simulink model "RoboNouMiChi"  (R2017b)
settings: Solver=VariableStepAuto  StartTime=0.0  StopTime=10.0  RelTol=1e-3
libraries: rptgenlib x2
settings Model: Creator=prave  LastModifiedBy=prave

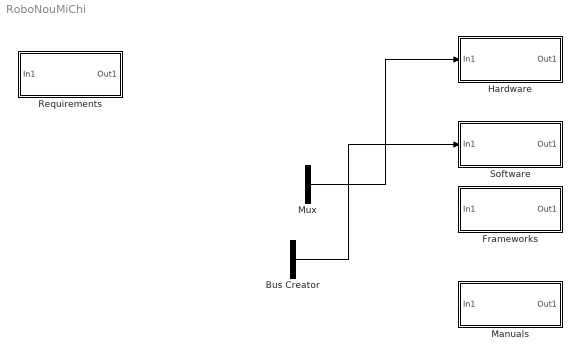
== system RoboNouMiChi ==
  Bus Creator : BusCreator  Inputs=2
  Frameworks : Subsystem  mask{Parameter1=0, Parameter2=on, Parameter3=on, Parameter4=on, Parameter5=on, Parameter6=on, Parameter7=on, Parameter8=on}
      mask prompts: Parameter1 "Heart"; Parameter2 "Heart beat estimator"; Parameter3 "Sensorless"; Parameter4 "Automotive"; Parameter5 "White balance estimator"; Parameter6 "Defect detector"; Parameter7 "Renesas"; Parameter8 "Fujitsu"
      mask DialogControl Container5 Prompt: Human
      mask DialogControl Container6 Prompt: Selection table
  Hardware : Subsystem  mask{Parameter1=0, Parameter2=on, Parameter3=on, Parameter4=on, Parameter5=on, Parameter6=on, Parameter7=on, Parameter8=on}
      mask prompts: Parameter1 "Frequency"; Parameter2 "Embedded DSP"; Parameter3 "Arm"; Parameter4 "FPGA"; Parameter5 "Cloud/Local PC"; Parameter6 "Cloud DSP"; Parameter7 "Renesas"; Parameter8 "Fujitsu"
      mask DialogControl Container5 Prompt: Hardware
      mask DialogControl Container6 Prompt: Selection table
  Manuals : Subsystem  mask{Parameter1=0, Parameter2=on, Parameter3=on, Parameter4=on, Parameter5=on, Parameter6=on, Parameter7=on, Parameter8=on}
      mask prompts: Parameter1 "Heart"; Parameter2 "Heart beat estimator"; Parameter3 "Sensorless"; Parameter4 "Automotive"; Parameter5 "White balance estimator"; Parameter6 "Defect detector"; Parameter7 "Renesas"; Parameter8 "Fujitsu"
      mask DialogControl Container5 Prompt: Human
      mask DialogControl Container6 Prompt: Selection table
  Mux : Mux  Inputs=2
  Requirements : Subsystem
  Software : Subsystem  mask{Parameter1=on, Parameter2=small, Parameter3=0}
      mask prompts: Parameter1 "Embed"; Parameter2 "C++"; Parameter3 "Frequency"
      mask TypeOptions Parameter2: small | big | medium
  wires:
  Mux/1 -> Hardware/1(In1)
  Bus Creator/1 -> Software/1(In1)

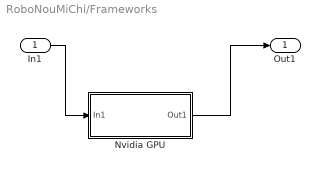
== system RoboNouMiChi/Frameworks ==
  In1 : Inport
  "Nvidia GPU " : Subsystem  TreatAsAtomicUnit=on
  Out1 : Outport
  wires:
  "Nvidia GPU "/1(Out1) -> Out1/1
  In1/1 -> "Nvidia GPU "/1(In1)

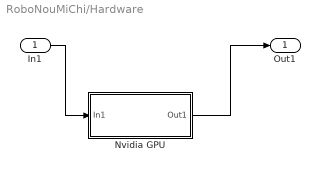
== system RoboNouMiChi/Hardware ==
  In1 : Inport
  "Nvidia GPU " : Subsystem  TreatAsAtomicUnit=on
  Out1 : Outport
  wires:
  In1/1 -> "Nvidia GPU "/1(In1)
  "Nvidia GPU "/1(Out1) -> Out1/1

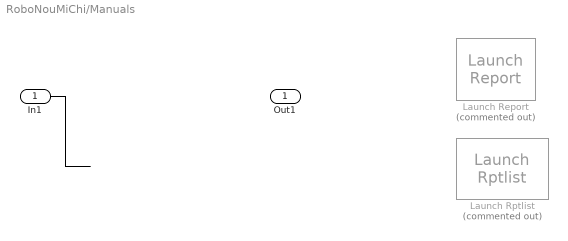
== system RoboNouMiChi/Manuals ==
  In1 : Inport
  Launch Report : rptgenlib/Launch Report  Tag=rptgen_sl  Description=Reports on the current system or model  Commented=on
      settings: SourceProductName=Simulink Report Generator  SourceProductBaseCode=SR
  Launch Rptlist : rptgenlib/Launch Rptlist  Tag=rptgen_sl  Description="This block launches the Report Generator Explorer. It lists all the setup files which the Report Generator can use to generate reports.  This GUI can also be used to set the current system's \"ReportName\" property."  Commented=on
      settings: SourceProductName=Simulink Report Generator  SourceProductBaseCode=SR
  Out1 : Outport
  wires:
  In1/1 -> ?
  ? -> Out1/1

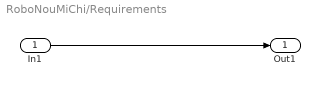
== system RoboNouMiChi/Requirements ==
  In1 : Inport
  Out1 : Outport
  wires:
  In1/1 -> Out1/1

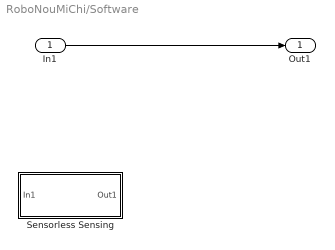
== system RoboNouMiChi/Software ==
  In1 : Inport
  "Sensorless Sensing " : Subsystem  TreatAsAtomicUnit=on
  Out1 : Outport
  wires:
  In1/1 -> Out1/1

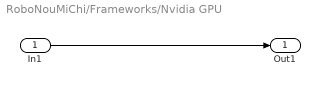
== system RoboNouMiChi/Frameworks/Nvidia GPU  ==
  In1 : Inport
  Out1 : Outport
  wires:
  In1/1 -> Out1/1

== system RoboNouMiChi/Hardware/Nvidia GPU  ==
  In1 : Inport
  Out1 : Outport
  wires:
  In1/1 -> Out1/1

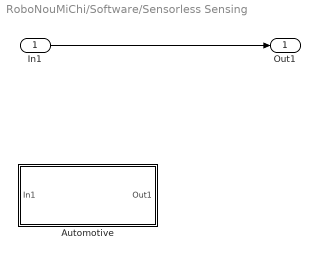
== system RoboNouMiChi/Software/Sensorless Sensing  ==
  In1 : Inport
  Automotive : Subsystem  TreatAsAtomicUnit=on
  Out1 : Outport
  wires:
  In1/1 -> Out1/1

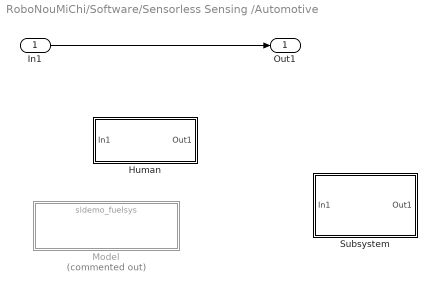
== system RoboNouMiChi/Software/Sensorless Sensing /Automotive ==
  In1 : Inport
  Human : Subsystem  TreatAsAtomicUnit=on
  Model : ModelReference  Commented=on  ModelNameDialog=sldemo_fuelsys.slx  SimulationMode=Normal  ModelReferenceVersion=1.738
  Subsystem : Subsystem  TreatAsAtomicUnit=on
  Out1 : Outport
  wires:
  In1/1 -> Out1/1

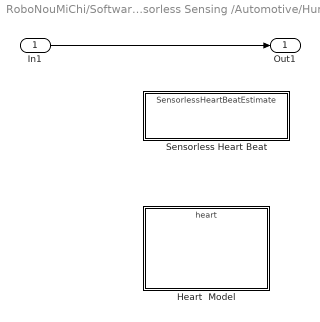
== system RoboNouMiChi/Software/Sensorless Sensing /Automotive/Human ==
  In1 : Inport
  Heart  Model : ModelReference  ModelNameDialog=heart.slx  SimulationMode=Normal  ModelReferenceVersion=1.14
      mask Display: image('genheartbeat.jpeg');
  Sensorless Heart Beat : ModelReference  ModelNameDialog=SensorlessHeartBeatEstimate.slx  SimulationMode=Normal  ModelReferenceVersion=1.3
  Out1 : Outport
  wires:
  In1/1 -> Out1/1

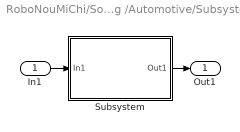
== system RoboNouMiChi/Software/Sensorless Sensing /Automotive/Subsystem ==
  In1 : Inport
  Subsystem : Subsystem
  Out1 : Outport
  wires:
  In1/1 -> Subsystem/1(In1)
  Subsystem/1(Out1) -> Out1/1

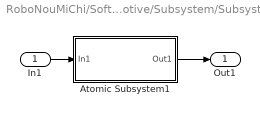
== system RoboNouMiChi/Software/Sensorless Sensing /Automotive/Subsystem/Subsystem ==
  In1 : Inport
  Atomic Subsystem1 : Subsystem  TreatAsAtomicUnit=on
  Out1 : Outport
  wires:
  Atomic Subsystem1/1(Out1) -> Out1/1
  In1/1 -> Atomic Subsystem1/1(In1)

== system RoboNouMiChi/Software/Sensorless Sensing /Automotive/Subsystem/Subsystem/Atomic Subsystem1 ==
  In1 : Inport
  Out1 : Outport
  wires:
  In1/1 -> Out1/1
